simulink model "MC_Chart"  (R2023b)
settings: Solver=FixedStepDiscrete  StartTime=0.0  StopTime=10.0  FixedStep=0.1  RelTol=1e-3  EnableMultiTasking=on
settings Model: Creator=diego  LastModifiedBy=diego
settings SolverCC: AlgebraicLoopSolver=TrustRegion  AutoInsertRateTranBlk=on
settings DataIOCC: LimitDataPoints=on
settings OptimizationCC: LifeSpan=inf
settings DebuggingCC: UnconnectedInputMsg=warning  UnconnectedOutputMsg=warning  UnconnectedLineMsg=warning  AllowSymbolicDim=off  SFUnexpectedBacktrackingDiag=warning  SFNoUnconditionalDefaultTransitionDiag=warning  SFExecutionAtInitializationDiag=none  ArithmeticOperatorsInVariantConditions=warning
settings ModelReferenceCC: EnableRefExpFcnMdlSchedulingChecks=on
settings SFSimCC: SimUseLocalCustomCode=off  CustomCodeUndefinedFunction=UseInterfaceOnly
settings RTWCC: RTWUseLocalCustomCode=off  DLArmComputeVersion=19.05
settings CodeAppCC: StateflowObjectComments=on
settings GRTTargetCC: TargetLangStandard=C89/C90 (ANSI)
settings ConfigComp: CovMetricSettings=dw  CovSaveCumulativeToWorkspaceVar=on  CovSaveSingleToWorkspaceVar=on  CovExternalEMLEnable=off  CovSFcnEnable=off

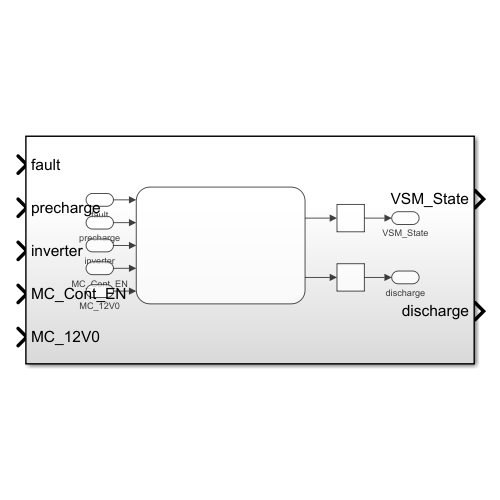
[thumbnail: Simulink's stored preview of the top-level diagram]
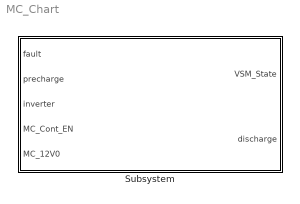
== system MC_Chart ==
  Subsystem : Subsystem

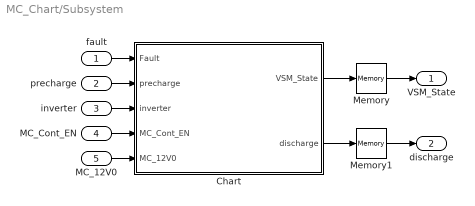
== system MC_Chart/Subsystem ==
  fault : Inport
  precharge : Inport  Port=2
  inverter : Inport  Port=3
  MC_Cont_EN : Inport  Port=4
  MC_12V0 : Inport  Port=5
  Chart : Stateflow chart  TreatAsAtomicUnit=on
  Memory : Memory
  Memory1 : Memory
  VSM_State : Outport
  discharge : Outport  Port=2
  wires:
  inverter/1 -> Chart/3(inverter)
  fault/1 -> Chart/1(Fault)
  Chart/2(discharge) -> Memory1/1
  MC_Cont_EN/1 -> Chart/4(MC_Cont_EN)
  precharge/1 -> Chart/2(precharge)
  Memory/1 -> VSM_State/1
  Chart/1(VSM_State) -> Memory/1
  Memory1/1 -> discharge/1
  MC_12V0/1 -> Chart/5(MC_12V0)

== stateflow chart MC_Chart/Subsystem/Chart ==
  state Start
    during:
    VSM_State = 0;
    state SubState
      state Power_Up
      state Init
      state POST
      state Load_EEPROM
      (default) -> Power_Up
      Power_Up -> Init
      Init -> Load_EEPROM
      Load_EEPROM -> POST
  state Precharge
    during:
    VSM_State = 1;
    after (2, sec);
    VSM_State = 2;
    after (2, sec);
    VSM_State = 3;
    after(2,sec);
    VSM_State = 4;
  state Wait
  state Fault
    during:
    VSM_State = 7;
  state Running
    during:
    VSM_State = 6;
  state Ready
    during:
    VSM_State = 5;
  state Discharge
    during:
    VSM_State = 7;
    state Discharge1
      during:
      discharge = 1;
    state Discharge2
      during:
      discharge = 2;
    state Discharge4
      during:
      discharge = 4;
    state Discharge3
      during:
      discharge = 3;
      after(9,sec)
    (default) -> Discharge1
    Discharge1 -> Discharge2 : [discharge == 1]
    Discharge2 -> Discharge3 : [RPM < 75]
    Discharge3 -> Discharge4 : [after(20,sec) && Voltage < 30]
  state Shutdown
    during:
    VSM_State = 14;
    discharge = 0;
  (default) -> Start
  Precharge -> Wait [order 2] : [precharge == 0]
  Start -> Precharge [order 1] : [precharge == 1]
  Precharge -> Fault [order 1] : [Fault == 1]
  Start -> Fault [order 2] : [Fault == 1]
  Wait -> Ready : [MC_Cont_EN == 1]
  Ready -> Fault [order 2] : after(100,sec)
  Ready -> Running [order 1] : [inverter == 1]
  Running -> Ready [order 1] : [inverter == 0 && MC_Cont_EN == 1]
  Fault -> Discharge
  Running -> Discharge [order 2] : [MC_Cont_EN == 0]
  Discharge -> Shutdown : [MC_12V0 == 0]
  data: Fault input; VSM_State output [0..14] =0; precharge input; inverter input; MC_Cont_EN input; discharge output =1; RPM local =0; Voltage local =0; MC_12V0 input
